simulink model "nlfilt"  (Simulink 6.3)
settings: Solver=FixedStepDiscrete  StartTime=0.0  StopTime=55  RelTol=1e-3
undefined symbols (not defined in the file or in its folder): TS
settings Model: LastModifiedBy=Kostas Tsakalis

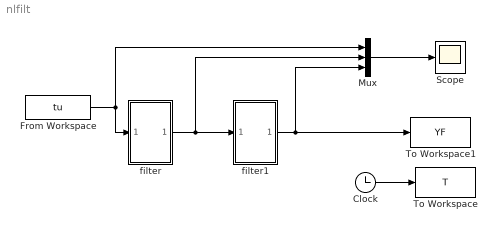
== system nlfilt ==
  Clock : Clock
      settings: Decimation=10
  From Workspace : FromWorkspace  VariableName=tu  SampleTime=0
  Mux : Mux  Inputs=3
  Scope : Scope
      settings: TimeRange=60  YMin=-200  YMax=400
  To Workspace : ToWorkspace  VariableName=T  SampleTime=-1  SaveFormat=Array
  To Workspace1 : ToWorkspace  VariableName=YF  SampleTime=-1  SaveFormat=Array
  filter : Subsystem  mask{emin=.5, emax=5, p=8, TS=TS}
      mask prompts: emin "error level to reject"; emax "error level to accept"; p "nonlin. power"; TS "sampling time"
  filter1 : Subsystem  mask{emin=.5, emax=5, p=8, TS=TS}
      mask prompts: emin "error level to reject"; emax "error level to accept"; p "nonlin. power"; TS "sampling time"
  wires:
  Clock/1 -> To Workspace/1
  From Workspace/1 -> filter/1(var), Mux/1
  filter/1(upd) -> filter1/1(var), Mux/2
  Mux/1 -> Scope/1
  filter1/1(upd) -> To Workspace1/1, Mux/3

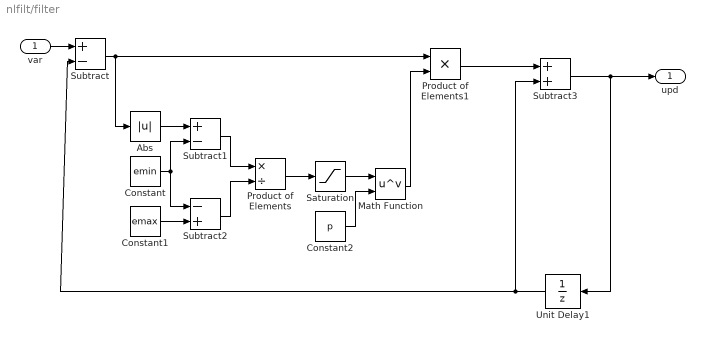
== system nlfilt/filter ==
  var : Inport
  Abs : Abs
  Constant : Constant  Value=emin
  Constant1 : Constant  Value=emax
  Constant2 : Constant  Value=p
  Math Function : Math  Operator=pow  SaturateOnIntegerOverflow=on
  Product of Elements : Product  Inputs=*/  OutScaling=2^-10
  Product of Elements1 : Product  OutScaling=2^-10
  Saturation : Saturate  UpperLimit=1  LowerLimit=0
  Subtract : Sum  Inputs=+-  OutScaling=2^-10
  Subtract1 : Sum  Inputs=+-  OutScaling=2^-10
  Subtract2 : Sum  Inputs=-+  OutScaling=2^-10
  Subtract3 : Sum  Inputs=2  OutScaling=2^-10
  Unit Delay1 : UnitDelay  Orientation=left  SampleTime=TS
  upd : Outport
  wires:
  Subtract/1 -> Abs/1, Product of Elements1/1
  Abs/1 -> Subtract1/1
  Constant/1 -> Subtract1/2, Subtract2/1
  Constant1/1 -> Subtract2/2
  Subtract2/1 -> Product of Elements/2
  Subtract1/1 -> Product of Elements/1
  Product of Elements/1 -> Saturation/1
  Saturation/1 -> Math Function/1
  Constant2/1 -> Math Function/2
  var/1 -> Subtract/1
  Math Function/1 -> Product of Elements1/2
  Product of Elements1/1 -> Subtract3/1
  Subtract3/1 -> upd/1, Unit Delay1/1
  Unit Delay1/1 -> Subtract3/2, Subtract/2

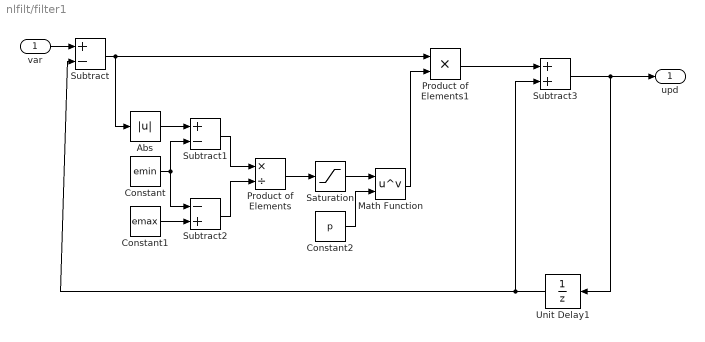
== system nlfilt/filter1 ==
  var : Inport
  Abs : Abs
  Constant : Constant  Value=emin
  Constant1 : Constant  Value=emax
  Constant2 : Constant  Value=p
  Math Function : Math  Operator=pow  SaturateOnIntegerOverflow=on
  Product of Elements : Product  Inputs=*/  OutScaling=2^-10
  Product of Elements1 : Product  OutScaling=2^-10
  Saturation : Saturate  UpperLimit=1  LowerLimit=0
  Subtract : Sum  Inputs=+-  OutScaling=2^-10
  Subtract1 : Sum  Inputs=+-  OutScaling=2^-10
  Subtract2 : Sum  Inputs=-+  OutScaling=2^-10
  Subtract3 : Sum  Inputs=2  OutScaling=2^-10
  Unit Delay1 : UnitDelay  Orientation=left  SampleTime=TS
  upd : Outport
  wires:
  Unit Delay1/1 -> Subtract/2, Subtract3/2
  Subtract3/1 -> Unit Delay1/1, upd/1
  Product of Elements1/1 -> Subtract3/1
  Math Function/1 -> Product of Elements1/2
  var/1 -> Subtract/1
  Constant2/1 -> Math Function/2
  Saturation/1 -> Math Function/1
  Product of Elements/1 -> Saturation/1
  Subtract1/1 -> Product of Elements/1
  Subtract2/1 -> Product of Elements/2
  Constant1/1 -> Subtract2/2
  Constant/1 -> Subtract2/1, Subtract1/2
  Abs/1 -> Subtract1/1
  Subtract/1 -> Product of Elements1/1, Abs/1
